simulink model "Parachute"  (R2018a)
settings: Solver=VariableStepAuto  StartTime=0.0  StopTime=4  RelTol=1e-4
values from neighbouring files (symbols this model uses):
  Bj = 10    [Main.m]
  Bp = 100    [Main.m]
  g = 9.807    [Main.m]
  Kr = 400    [Main.m]
  Mj = 60    [Main.m]
  Mp = 10    [Main.m]
  V0j = 20    [Main.m]
  V0p = 20    [Main.m]
  X0j = 0    [Main.m]
  X0p = 0    [Main.m]
settings Model: Creator=Eduardo  LastModifiedBy=Eduardo

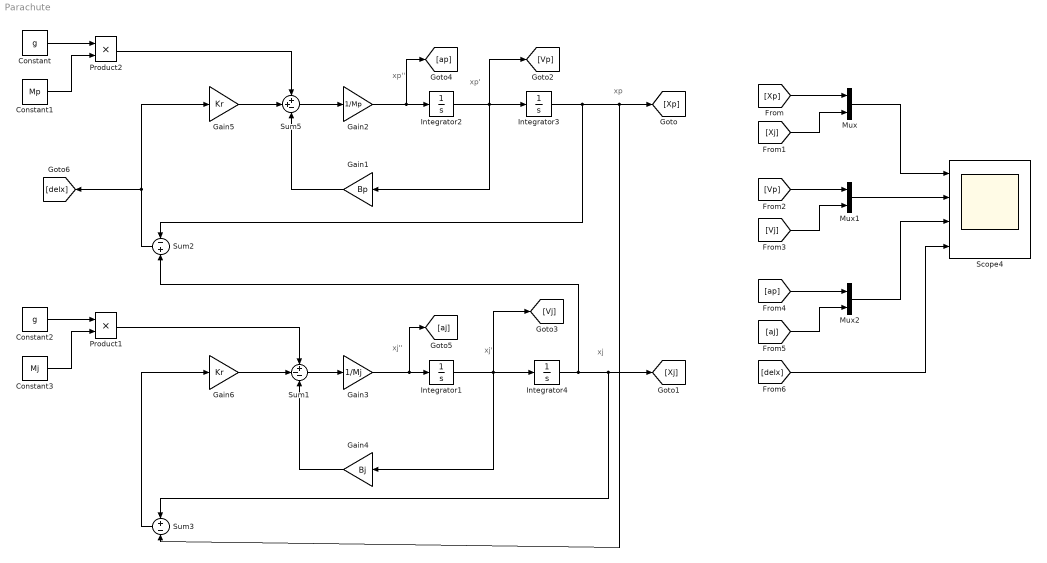
== system Parachute ==
  note: xp
  note: xj
  note: xj'
  note: xj''
  note: xp'
  note: xp''
  Constant : Constant  Value=g
  Constant1 : Constant  Value=Mp
  Constant2 : Constant  Value=g
  Constant3 : Constant  Value=Mj
  Gain1 : Gain  Gain=Bp
  Gain2 : Gain  Gain=1/Mp
  Gain3 : Gain  Gain=1/Mj
  Gain4 : Gain  Gain=Bj
  Gain5 : Gain  Gain=Kr
  Gain6 : Gain  Gain=Kr
  Integrator1 : Integrator  InitialCondition=V0j
  Integrator2 : Integrator  InitialCondition=V0p
  Integrator3 : Integrator  InitialCondition=X0p
  Integrator4 : Integrator  InitialCondition=X0j
  Mux : Mux  Inputs=2
  Mux1 : Mux  Inputs=2
  Mux2 : Mux  Inputs=2
  Product1 : Product
  Product2 : Product
  Scope4 : Scope  NumInputPorts=4
  Sum1 : Sum  Inputs=+--
  Sum2 : Sum  Inputs=-+
  Sum3 : Sum  Inputs=+-
  Sum5 : Sum  Inputs=++-
  wires:
  Constant1/1 -> Product2/2
  Constant/1 -> Product2/1
  Product2/1 -> Sum5/1
  Sum5/1 -> Gain2/1
  Gain2/1 -> [ap], Integrator2/1
  Integrator2/1 -> [Vp], Integrator3/1, Gain1/1
  Gain1/1 -> Sum5/3
  Integrator3/1 -> [Xp], Sum3/2, Sum2/1
  Constant2/1 -> Product1/1
  Constant3/1 -> Product1/2
  Product1/1 -> Sum1/1
  Sum1/1 -> Gain3/1
  Gain3/1 -> [aj], Integrator1/1
  Gain4/1 -> Sum1/3
  Gain5/1 -> Sum5/2
  Integrator4/1 -> [Xj], Sum3/1, Sum2/2
  Sum2/1 -> [delx], Gain5/1
  Gain6/1 -> Sum1/2
  Sum3/1 -> Gain6/1
  Integrator1/1 -> [Vj], Gain4/1, Integrator4/1
  [Xp] -> Mux/1
  [Xj] -> Mux/2
  [ap] -> Mux2/1
  [aj] -> Mux2/2
  [Vp] -> Mux1/1
  [Vj] -> Mux1/2
  Mux/1 -> Scope4/1
  Mux1/1 -> Scope4/2
  Mux2/1 -> Scope4/3
  [delx] -> Scope4/4
